simulink model "ES200A_CurrMeas"  (R2013b)
settings: Solver=FixedStepDiscrete  SolverMode=SingleTasking  StartTime=0.0  StopTime=1  FixedStep=0.000125  RelTol=1e-3
values from neighbouring files (symbols this model uses):
  ARCHGLBPRM_2PI_ULS_F32 = DataDict.Constant    [ES200A_CurrMeas_DataDict.m]
  CurrMeasEolGainMax = DataDict.Calibration    [ES200A_CurrMeas_DataDict.m]
  CurrMeasEolGainMin = DataDict.Calibration    [ES200A_CurrMeas_DataDict.m]
  CurrMeasEolGainNrOfSample = DataDict.Calibration    [ES200A_CurrMeas_DataDict.m]
  CurrMeasEolGainNumer = DataDict.Calibration    [ES200A_CurrMeas_DataDict.m]
  CurrMeasEolMaxMotVel = DataDict.Calibration    [ES200A_CurrMeas_DataDict.m]
  CurrMeasEolOffsHiBrdgVltgMin = DataDict.Calibration    [ES200A_CurrMeas_DataDict.m]
  CurrMeasEolOffsHiCmuOffs = DataDict.Calibration    [ES200A_CurrMeas_DataDict.m]
  CurrMeasEolOffsLoCmuOffs = DataDict.Calibration    [ES200A_CurrMeas_DataDict.m]
  CurrMeasEolOffsMax = DataDict.Calibration    [ES200A_CurrMeas_DataDict.m]
  CurrMeasEolOffsMin = DataDict.Calibration    [ES200A_CurrMeas_DataDict.m]
  CurrMeasEolOffsNrOfSample = DataDict.Calibration    [ES200A_CurrMeas_DataDict.m]
  CurrMeasEolTranCntrThd = DataDict.Calibration    [ES200A_CurrMeas_DataDict.m]
  CurrMeasMinRqrdPhaOnTi = DataDict.Calibration    [ES200A_CurrMeas_DataDict.m]
  CurrMeasMotAgCompuDly = DataDict.Calibration    [ES200A_CurrMeas_DataDict.m]
  CurrMeasMotCurrAdcVlyWrmIninMax = DataDict.Calibration    [ES200A_CurrMeas_DataDict.m]
  CurrMeasMotCurrAdcVlyWrmIninMin = DataDict.Calibration    [ES200A_CurrMeas_DataDict.m]
  CurrMeasNtc0x05DFailStep = DataDict.Calibration    [ES200A_CurrMeas_DataDict.m]
  CurrMeasNtc0x05DPassStep = DataDict.Calibration    [ES200A_CurrMeas_DataDict.m]
  CurrMeasNtc0x06DFailStep = DataDict.Calibration    [ES200A_CurrMeas_DataDict.m]
  CurrMeasNtc0x06DPassStep = DataDict.Calibration    [ES200A_CurrMeas_DataDict.m]
  DEGREES30_MOTRAD_F32 = DataDict.Constant    [ES200A_CurrMeas_DataDict.m]
  DIFOFFSRNGCHKMAX_VOLT_F32 = DataDict.Constant    [ES200A_CurrMeas_DataDict.m]
  ELECGLBPRM_IVTRCNT_CNT_U08 = DataDict.ConfigParam    [ES200A_CurrMeas_DataDict.m]
  ELECGLBPRM_STRTUPSTCURRMEASWRMININTESTSTRT_CNT_U08 = DataDict.Constant    [ES200A_CurrMeas_DataDict.m]
  FLTINJ_CURRMEAS_MOTCURRCORRDA = DataDict.Constant    [ES200A_CurrMeas_DataDict.m]
  FLTINJ_CURRMEAS_MOTCURRCORRDD = DataDict.Constant    [ES200A_CurrMeas_DataDict.m]
  FLTINJ_CURRMEAS_TESTOK = DataDict.Constant    [ES200A_CurrMeas_DataDict.m]
  MAXCURRCORRD_AMPR_F32 = DataDict.Constant    [ES200A_CurrMeas_DataDict.m]
  PhaABCMeasdOutOfRng = DataDict.NTC    [ES200A_CurrMeas_DataDict.m]
  PhaDEFMeasOutOfRng = DataDict.NTC    [ES200A_CurrMeas_DataDict.m]
  SysGlbPrmMotPoleCnt = DataDict.ImprtdCal    [ES200A_CurrMeas_DataDict.m]
libraries: simulink x10, FixdToFloat x1
(part 3 of 7)

== stateflow chart ES200A_CurrMeas/CurrMeas/CurrMeasPer1/Offset Calibration/Offset State Machine ==
  note: EolOffsSts
      |
      | 0 = Not Started
      | 1 = Started/In Process
      | 2 = Successful
      | 4  = Phase A, B, C EOL Calculated Gains are Out Of Range
      | 8  = Phase D, E, F EOL Calculated Gains are Out Of Range
      | 12 = Phase A, B, C, D, E, F EOL Calculated Gains are Out Of Range
      | 16  = VehSpd, VehSpdVld, condition not met
      | 32  = MotVelMrf condition not met
      | 64 = DiagcStsIvtr1Inactv and DiagcStsIvtr1Inactv both TRUE
  note: EolOffsOutOfRng = NTCNR_0X1EC
      | Parameters:
      |        Bit0Descr = 1 = 0000 0001 = Phase A, B, C EOL Calculated Offsets are Out Of Range
      |        Bit1Descr = 2 = 0000 0010 = Phase D, E, F EOL Calculated Offsets are Out Of Range
      |        Bit0Descr | Bit1Descr = 3 = 0000 0011 = Phase A, B, C, D, E, F EOL Calculated Offsets are Out Of Range
      |        Bit2Descr = 4 = 0000 0100 = VehSpd, VehSpdVld, condition not met
      |        Bit3Descr = 8 = 0000 1000 = MotVelMrf condition not met
      |        Bit3Descr = 16 = 0001 0000 = DiagcStsIvtr1Inactv and DiagcStsIvtr1Inactv both TRUE
  state MotCurrNtcSet = SetNtcSts(NTCNr,ParamBit,NTCSts,NTCDebStep) [function]
  note: EolOffsSts
      |
      | 0 = Not Started
      | 1 = Started/In Process
      | 2 = Successful
      | 4  = Phase A, B, C EOL Calculated Gains are Out Of Range
      | 8  = Phase D, E, F EOL Calculated Gains are Out Of Range
      | 12 = Phase A, B, C, D, E, F EOL Calculated Gains are Out Of Range
      | 16  = VehSpd, VehSpdVld, condition not met
      | 32  = MotVelMrf condition not met
      | 64 = DiagcStsIvtr1Inactv and DiagcStsIvtr1Inactv both TRUE
  note: EolOffsOutOfRng = NTCNR_0X1EC
      | Parameters:
      |        Bit0Descr = 1 = 0000 0001 = Phase A, B, C EOL Calculated Offsets are Out Of Range
      |        Bit1Descr = 2 = 0000 0010 = Phase D, E, F EOL Calculated Offsets are Out Of Range
      |
      |        Bit0Descr | Bit1Descr = 3 = 0000 0011 = Phase A, B, C, D, E, F EOL Calculated Offsets are Out Of Range
      |
      |        Bit2Descr = 4 = 0000 0100 = VehSpd, VehSpdVld, condition not met
      |        Bit3Descr = 8 = 0000 1000 = MotVelMrf condition not met
      |        Bit3Descr = 16 = 0001 0000 = DiagcStsIvtr1Inactv and DiagcStsIvtr1Inactv both TRUE
  state WrNvm [function]
  (default) -> (junction 307) : {EolOffsSts = EolOffsStsPrev;}
  (junction 307) -> (junction 233) [order 2] : {EolOffsSts = EolOffsStsPrev;}
  (junction 307) -> (junction 188) [order 1] : [EolOffsSts == 1]
  (junction 188) -> (junction 452) [order 1] : [(VehSpd <= ARCHGLBPRM_FLOATZEROTHD_ULS_F32 )...
      |  && (VehSpdVld == 1)]
  (junction 452) -> (junction 186) [order 1] : [(abs(MotVelMrf) <= CurrMeasEolMaxMotVel)]
  (junction 186) -> (junction 245) [order 2]
  (junction 245) -> (junction 263) [order 2]
  (junction 263) -> (junction 284) [order 2]
  (junction 284) -> (junction 294) [order 2]
  (junction 452) -> (junction 455) [order 2] : {CurrMeasMotCurrEolCalSt = MotCurrEolCalSt2.MCECS_CMDSAFEST;
      | MotCurrNtcSet = SetNtcSts(EolOffsOutOfRng, 8, 1, 0);
      | EolOffsSts = 32;}
  (junction 188) -> (junction 233) [order 2] : {CurrMeasMotCurrEolCalSt = MotCurrEolCalSt2.MCECS_CMDSAFEST;
      | MotCurrNtcSet = SetNtcSts(EolOffsOutOfRng, 4, 1, 0);
      | EolOffsSts = 16;}
  (junction 186) -> (junction 194) [order 1] : [(CurrMeasMotCurrEolCalStPrev == 0) || (CurrMeasMotCurrEolCalStPrev == 1)]
      | {CurrMeasMotCurrEolCalSt = MotCurrEolCalSt2.MCECS_OFFSCMDHI;}
  (junction 245) -> (junction 238) [order 1] : [CurrMeasMotCurrEolCalStPrev == MotCurrEolCalSt2.MCECS_OFFSCMDLO]
  (junction 263) -> (junction 256) [order 1] : [CurrMeasMotCurrEolCalStPrev == MotCurrEolCalSt2.MCECS_OFFSCMDZERO]
  (junction 284) -> (junction 395) [order 1] : [CurrMeasMotCurrEolCalStPrev == MotCurrEolCalSt2.MCECS_OFFSCMDEND && MotCurrEolOffsProcFlg != 1]
  (junction 294) -> (junction 295)
  (junction 395) -> (junction 414) [order 2] : {OffsRngChkABC = 1;}
  (junction 395) -> (junction 281) [order 1] : [DiagcStsIvtr1Inactv == 0]
  (junction 281) -> (junction 418) [order 2]
  (junction 418) -> (junction 434) : {OffsFltParam = 1;
      | OffsRngChkABC = 0;}
  (junction 281) -> (junction 414) [order 1] : [((MotCurrOffsHiAvrgA >= CurrMeasEolOffsMin) && (MotCurrOffsHiAvrgA <= CurrMeasEolOffsMax)) &&...
      | ((MotCurrOffsHiAvrgB >= CurrMeasEolOffsMin) && (MotCurrOffsHiAvrgB <= CurrMeasEolOffsMax)) &&...
      | ((MotCurrOffsHiAvrgC >= CurrMeasEolOffsMin) && (MotCurrOffsHiAvrgC <= CurrMeasEolOffsMax)) &&...
      | ((MotCurrOffsLoAvrgA >= CurrMeasEolOffsMin) && (MotCurrOffsLoAvrgA <= CurrMeasEolOffsMax)) &&...
      | ((MotCurrOffsLoAvrgB >= CurrMeasEolOffsMin) && (MotCurrOffsLoAvrgB <= CurrMeasEolOffsMax)) &&...
      | ((MotCurrOffsLoAvrgC >= CurrMeasEolOffsMin) && (MotCurrOffsLoAvrgC <= CurrMeasEolOffsMax))]
      |
      | {OffsRngChkABC = 1;}
  (junction 194) -> (junction 204) [order 2] : {CurrMeasEolTranCntr = CurrMeasEolTranCntrPrev + 1;}
  (junction 238) -> (junction 249) [order 2] : {CurrMeasEolTranCntr = CurrMeasEolTranCntrPrev + 1;}
  (junction 256) -> (junction 261) [order 2] : {CurrMeasEolTranCntr = CurrMeasEolTranCntrPrev + 1;}
  (junction 194) -> (junction 200) [order 1] : [CurrMeasEolTranCntr == CurrMeasEolTranCntrThd]
      |
      | {CurrMeasMotCurrSumA = CurrMeasMotCurrSumAPrev + MotCurrAdcVlyA;
      | CurrMeasMotCurrSumB = CurrMeasMotCurrSumBPrev + MotCurrAdcVlyB;
      | CurrMeasMotCurrSumC = CurrMeasMotCurrSumCPrev + MotCurrAdcVlyC;
      | CurrMeasMotCurrSumD = CurrMeasMotCurrSumDPrev + MotCurrAdcVlyD;
      | CurrMeasMotCurrSumE = CurrMeasMotCurrSumEPrev + MotCurrAdcVlyE;
      | CurrMeasMotCurrSumF = CurrMeasMotCurrSumFPrev + MotCurrAdcVlyF;
      | CurrMeasBrdgVltgSum = CurrMeasBrdgVltgSumPrev + BrdgVltg;
      |
      | CurrMeasEolAvrgCntr = CurrMeasEolAvrgCntrPrev + 1;}
  (junction 238) -> (junction 241) [order 1] : [CurrMeasEolTranCntr == CurrMeasEolTranCntrThd]
      |
      | {CurrMeasMotCurrSumA = CurrMeasMotCurrSumAPrev + MotCurrAdcVlyA;
      | CurrMeasMotCurrSumB = CurrMeasMotCurrSumBPrev + MotCurrAdcVlyB;
      | CurrMeasMotCurrSumC = CurrMeasMotCurrSumCPrev + MotCurrAdcVlyC;
      | CurrMeasMotCurrSumD = CurrMeasMotCurrSumDPrev + MotCurrAdcVlyD;
      | CurrMeasMotCurrSumE = CurrMeasMotCurrSumEPrev + MotCurrAdcVlyE;
      | CurrMeasMotCurrSumF = CurrMeasMotCurrSumFPrev + MotCurrAdcVlyF;
      |
      |
      | CurrMeasEolAvrgCntr = CurrMeasEolAvrgCntrPrev + 1;}
  (junction 256) -> (junction 254) [order 1] : [CurrMeasEolTranCntr == CurrMeasEolTranCntrThd]
      |
      | {CurrMeasMotCurrSumA = CurrMeasMotCurrSumAPrev + MotCurrAdcVlyA;
      | CurrMeasMotCurrSumB = CurrMeasMotCurrSumBPrev + MotCurrAdcVlyB;
      | CurrMeasMotCurrSumC = CurrMeasMotCurrSumCPrev + MotCurrAdcVlyC;
      | CurrMeasMotCurrSumD = CurrMeasMotCurrSumDPrev + MotCurrAdcVlyD;
      | CurrMeasMotCurrSumE = CurrMeasMotCurrSumEPrev + MotCurrAdcVlyE;
      | CurrMeasMotCurrSumF = CurrMeasMotCurrSumFPrev + MotCurrAdcVlyF;
      |
      |
      | CurrMeasEolAvrgCntr = CurrMeasEolAvrgCntrPrev + 1;}
  (junction 434) -> (junction 414)
  (junction 414) -> (junction 368)
  (junction 368) -> (junction 283) [order 2] : {OffsRngChkDEF = 1;}
  (junction 368) -> (junction 398) [order 1] : [DiagcStsIvtr2Inactv == 0 && ELECGLBPRM_IVTRCNT_CNT_U08 == 2]
  (junction 398) -> (junction 421) [order 2]
  (junction 421) -> (junction 436) : {OffsFltParam = OffsFltParam + 2
      | OffsRngChkDEF = 0;}
  (junction 398) -> (junction 283) [order 1] : [((MotCurrOffsHiAvrgD >= CurrMeasEolOffsMin) && (MotCurrOffsHiAvrgD <= CurrMeasEolOffsMax)) &&...
      | ((MotCurrOffsHiAvrgE >= CurrMeasEolOffsMin) && (MotCurrOffsHiAvrgE <= CurrMeasEolOffsMax)) &&...
      | ((MotCurrOffsHiAvrgF >= CurrMeasEolOffsMin) && (MotCurrOffsHiAvrgF <= CurrMeasEolOffsMax)) &&...
      | ((MotCurrOffsLoAvrgD >= CurrMeasEolOffsMin) && (MotCurrOffsLoAvrgD <= CurrMeasEolOffsMax)) &&...
      | ((MotCurrOffsLoAvrgE >= CurrMeasEolOffsMin) && (MotCurrOffsLoAvrgE <= CurrMeasEolOffsMax)) &&...
      | ((MotCurrOffsLoAvrgF >= CurrMeasEolOffsMin) && (MotCurrOffsLoAvrgF <= CurrMeasEolOffsMax))]
      |
      | {OffsRngChkDEF = 1;}
  (junction 436) -> (junction 283)
  (junction 283) -> (junction 439)
  (junction 200) -> (junction 204) [order 2]
  (junction 241) -> (junction 249) [order 2]
  (junction 254) -> (junction 261) [order 2]
  (junction 200) -> (junction 204) [order 1] : [CurrMeasEolAvrgCntr == CurrMeasEolOffsNrOfSample]
      |
      | {MotCurrOffsHiAvrgA = CurrMeasMotCurrSumA / CurrMeasEolOffsNrOfSample;
      | MotCurrOffsHiAvrgB = CurrMeasMotCurrSumB / CurrMeasEolOffsNrOfSample;
      | MotCurrOffsHiAvrgC = CurrMeasMotCurrSumC / CurrMeasEolOffsNrOfSample;
      | MotCurrOffsHiAvrgD = CurrMeasMotCurrSumD / CurrMeasEolOffsNrOfSample;
      | MotCurrOffsHiAvrgE = CurrMeasMotCurrSumE / CurrMeasEolOffsNrOfSample;
      | MotCurrOffsHiAvrgF = CurrMeasMotCurrSumF / CurrMeasEolOffsNrOfSample;
      | BrdgVltgAvrg  = CurrMeasBrdgVltgSum / CurrMeasEolOffsNrOfSample;
      | MotCurrEolOffsHiBrdgVltg = BrdgVltgAvrg * (CurrMeasEolOffsHiCmuOffs...
      |  - CurrMeasEolOffsLoCmuOffs);
      |
      | CurrMeasMotCurrEolCalSt = MotCurrEolCalSt2.MCECS_OFFSCMDLO;
      |
      | CurrMeasEolAvrgCntr = 0;
      | CurrMeasEolTranCntr = 0;
      |
      | CurrMeasMotCurrSumA = 0;
      | CurrMeasMotCurrSumB = 0;
      | CurrMeasMotCurrSumC = 0;
      | CurrMeasMotCurrSumD = 0;
      | CurrMeasMotCurrSumE = 0;
      | CurrMeasMotCurrSumF = 0;}
  (junction 241) -> (junction 249) [order 1] : [CurrMeasEolAvrgCntr == CurrMeasEolOffsNrOfSample]
      |
      | {MotCurrOffsLoAvrgA = CurrMeasMotCurrSumA / CurrMeasEolOffsNrOfSample;
      | MotCurrOffsLoAvrgB = CurrMeasMotCurrSumB / CurrMeasEolOffsNrOfSample;
      | MotCurrOffsLoAvrgC = CurrMeasMotCurrSumC / CurrMeasEolOffsNrOfSample;
      | MotCurrOffsLoAvrgD = CurrMeasMotCurrSumD / CurrMeasEolOffsNrOfSample;
      | MotCurrOffsLoAvrgE = CurrMeasMotCurrSumE / CurrMeasEolOffsNrOfSample;
      | MotCurrOffsLoAvrgF = CurrMeasMotCurrSumF / CurrMeasEolOffsNrOfSample;
      |
      |
      |
      |
      | CurrMeasMotCurrEolCalSt = MotCurrEolCalSt2.MCECS_OFFSCMDZERO;
      |
      | CurrMeasEolAvrgCntr = 0;
      | CurrMeasEolTranCntr = 0;
      |
      | CurrMeasMotCurrSumA = 0;
      | CurrMeasMotCurrSumB = 0;
      | CurrMeasMotCurrSumC = 0;
      | CurrMeasMotCurrSumD = 0;
      | CurrMeasMotCurrSumE = 0;
      | CurrMeasMotCurrSumF = 0;}
  (junction 254) -> (junction 261) [order 1] : [CurrMeasEolAvrgCntr == CurrMeasEolOffsNrOfSample]
      |
      | {MotCurrOffsZeroAvrgA = CurrMeasMotCurrSumA / CurrMeasEolOffsNrOfSample;
      | MotCurrOffsZeroAvrgB = CurrMeasMotCurrSumB / CurrMeasEolOffsNrOfSample;
      | MotCurrOffsZeroAvrgC = CurrMeasMotCurrSumC / CurrMeasEolOffsNrOfSample;
      | MotCurrOffsZeroAvrgD = CurrMeasMotCurrSumD / CurrMeasEolOffsNrOfSample;
      | MotCurrOffsZeroAvrgE = CurrMeasMotCurrSumE / CurrMeasEolOffsNrOfSample;
      | MotCurrOffsZeroAvrgF = CurrMeasMotCurrSumF / CurrMeasEolOffsNrOfSample;
      |
      |
      |
      |
      | CurrMeasMotCurrEolCalSt = MotCurrEolCalSt2.MCECS_OFFSCMDEND;
      |
      | CurrMeasEolAvrgCntr = 0;
      | CurrMeasEolTranCntr = 0;
      |
      | CurrMeasMotCurrSumA = 0;
      | CurrMeasMotCurrSumB = 0;
      | CurrMeasMotCurrSumC = 0;
      | CurrMeasMotCurrSumD = 0;
      | CurrMeasMotCurrSumE = 0;
      | CurrMeasMotCurrSumF = 0;}
  (junction 439) -> (junction 441) [order 2]
  (junction 441) -> (junction 417) : {
      | CurrMeasMotCurrEolCalSt = MotCurrEolCalSt2.MCECS_CMDSAFEST
      | MotCurrNtcSet = SetNtcSts(EolOffsOutOfRng, OffsFltParam, 1, 0);
      | EolOffsSts = OffsFltParam * 4;
      | CurrMeasEolAvrgCntr = 0;
      | CurrMeasEolTranCntr = 0;
      | }
  (junction 439) -> (junction 443) [order 1] : [OffsRngChkABC == 1 && OffsRngChkDEF == 1]
      | {
      | CurrMeasMotCurrEolCalSt = MotCurrEolCalSt2.MCECS_OFFSCMDEND;
      | CurrMeasEolAvrgCntr = 0;
      | CurrMeasEolTranCntr = 0;
      | }
  (junction 443) -> (junction 445) [order 2]
  (junction 445) -> (junction 422) : {
      | MotCurrNtcSet = SetNtcSts(EolOffsOutOfRng, 16, 1, 0);
      | EolOffsSts = 64;
      | CurrMeasMotCurrEolCalSt = MotCurrEolCalSt2.MCECS_CMDSAFEST;
      | }
  (junction 443) -> (junction 288) [order 1] : [(DiagcStsIvtr1Inactv == 0 || DiagcStsIvtr2Inactv == 0)]
      | {
      | MotCurrNtcSet = SetNtcSts(EolOffsOutOfRng, 0, 0, 0);
      | WrNvm();
      | MotCurrEolOffsProcFlg = 1;
      | EolOffsSts = 2;
      | }
  (junction 233) -> (junction 455)
  (junction 455) -> (junction 204)
  (junction 204) -> (junction 249)
  (junction 249) -> (junction 261)
  (junction 261) -> (junction 417)
  (junction 417) -> (junction 422)
  (junction 422) -> (junction 288)
  (junction 295) -> (junction 288)
  (junction 288) -> (junction 428)
  data: NTCNr function_input; ParamBit function_input; MotCurrNtcSet function_output; NTCSts function_input; NTCDebStep function_input; CurrMeasMotCurrEolCalSt output Enum: MotCurrEolCalSt2; EolOffsSts output uint8; MotCurrAdcVlyA input; MotCurrAdcVlyB input; MotCurrAdcVlyC input; MotCurrAdcVlyD input; MotCurrAdcVlyE input; MotCurrAdcVlyF input; BrdgVltg input; CurrMeasEolOffsNrOfSample input; CurrMeasEolOffsHiCmuOffs input; CurrMeasEolOffsLoCmuOffs input; CurrMeasEolOffsMax input; CurrMeasEolOffsMin input; BrdgVltgAvrg local double; BrdgVltgSum local double; MotCurrOffAvrgCntr local single; MotCurrSumHiA local single; MotCurrSumHiB local single; MotCurrSumHiC local single; MotCurrSumLoA local single; MotCurrSumLoB local single; MotCurrSumLoC local single; MotCurrSumZeroA local single; MotCurrSumZeroB local single; MotCurrSumZeroC local single; MotCurrOffsZeroAvrgA output single; MotCurrOffsZeroAvrgB output single; MotCurrOffsZeroAvrgC output single; MotCurrOffsZeroAvrgD output single; MotCurrOffsZeroAvrgE output single; MotCurrOffsZeroAvrgF output single; MotCurrEolOffsProcFlg output boolean; MotCurrEolOffsHiBrdgVltg output single; MotCurrOffsHiAvrgA output single; MotCurrOffsHiAvrgB output single; MotCurrOffsHiAvrgC output single; MotCurrOffsHiAvrgD output single; MotCurrOffsHiAvrgE output single; MotCurrOffsHiAvrgF output single; MotCurrSumHiD local single; MotCurrSumHiE local single; MotCurrSumHiF local single; MotCurrSumLoD local single; MotCurrSumLoE local single; MotCurrSumLoF local single; MotCurrSumZeroD local single; MotCurrSumZeroE local single; MotCurrSumZeroF local single; MotCurrOffsLoAvrgA output single; MotCurrNtcSet local single; NTC1EC constant single; CurrMeasEolMaxMotVel input; CurrMeasEolTranCntrThd input; MotVelMrf input; VehSpd input; VehSpdVld input; CurrMeasMotCurrEolCalStPrev input; EolOffsStsPrev input; ELECGLBPRM_IVTRCNT_CNT_U08 input; DiagcStsIvtr1Inactv input; DiagcStsIvtr2Inactv input; MotCurrOffsLoAvrgB output single; MotCurrOffsLoAvrgC output single; MotCurrOffsLoAvrgD output single; MotCurrOffsLoAvrgE output single; MotCurrOffsLoAvrgF output single; CurrMeasBrdgVltgSumPrev input; CurrMeasMotCurrSumAPrev input single; CurrMeasMotCurrSumBPrev input; CurrMeasMotCurrSumCPrev input; CurrMeasMotCurrSumDPrev input; CurrMeasMotCurrSumEPrev input; CurrMeasMotCurrSumFPrev input; CurrMeasBrdgVltgSum output single; CurrMeasMotCurrSumA output single; CurrMeasMotCurrSumB output single; CurrMeasMotCurrSumC output single; CurrMeasMotCurrSumD output single; CurrMeasMotCurrSumE output single; CurrMeasMotCurrSumF output single; CurrMeasEolTranCntrPrev input; CurrMeasEolAvrgCntrPrev input; CurrMeasEolTranCntr output uint8; CurrMeasEolAvrgCntr output uint16; EolOffsOutOfRng constant double; OffsRngChkABC local double; OffsRngChkDEF local double; OffsFltParam local double; ARCHGLBPRM_FLOATZEROTHD_ULS_F32 parameter

== system ES200A_CurrMeas/CurrMeas/CurrMeasEolOffsStsReq ==
  function : TriggerPort  TriggerType=function-call
  CopyRight2 : Subsystem  Description=|  mask(Copyright Information){none=on}
      | Copyright info block.                                               
      |                                                                     
      | Place copyright information at the top of every subsystem in design.
      mask prompts: none "No parameters"
      mask help: Place copyright information at the top of every subsystem in design.
      mask Display:
      | NxtrConf = 'Nexteer Confidential';
      | 
      | sys = bdroot; %handle for the current model ("system")
      | first = get_param(sys,'Created');
      | first = first(end-3:end);  %year is last four digits
      | 
      | last = get_param(sys,'LastModifiedDate');
      | if isempty(last)
      |     last = datestr(now,'yyyy');
      | else
      |     last = last(end-3:end);
      | end
      | 
      | if strcmp(first,last)
      |     fprintf('%s -- Copyright %s Nexteer',NxtrConf,first)
      | else
      |     fprintf('%s -- %s%s- %s Nexteer',NxtrConf,char(169),first,last)
      | end
  EolOffsSts : DataStoreRead  DataStoreName=EolOffsSts  DataStoreElements=EolOffsSts
  CurrMeasEolOffsSt : Outport
  wires:
  EolOffsSts/1 -> CurrMeasEolOffsSt/1

== system ES200A_CurrMeas/CurrMeas/CurrMeasGainReadReq ==
  function : TriggerPort
  CopyRight2 : Subsystem  Description=|  mask(Copyright Information){none=on}
      | Copyright info block.                                               
      |                                                                     
      | Place copyright information at the top of every subsystem in design.
      mask prompts: none "No parameters"
      mask help: Place copyright information at the top of every subsystem in design.
      mask Display:
      | NxtrConf = 'Nexteer Confidential';
      | 
      | sys = bdroot; %handle for the current model ("system")
      | first = get_param(sys,'Created');
      | first = first(end-3:end);  %year is last four digits
      | 
      | last = get_param(sys,'LastModifiedDate');
      | if isempty(last)
      |     last = datestr(now,'yyyy');
      | else
      |     last = last(end-3:end);
      | end
      | 
      | if strcmp(first,last)
      |     fprintf('%s -- Copyright %s Nexteer',NxtrConf,first)
      | else
      |     fprintf('%s -- %s%s- %s Nexteer',NxtrConf,char(169),first,last)
      | end
  CurrMeasEolGainCalSet : DataStoreRead  DataStoreName=CurrMeasEolGainCalSet  DataStoreElements=CurrMeasEolGainCalSet.CurrMeasMotCurrEolGainA#CurrMeasEolGainCalSet.CurrMeasMotCurrEolGainB#CurrMeasEolGainCalSet.CurrMeasMotCurrEolGainC#CurrMeasEolGainCalSet.CurrMeasMotCurrEolGainD#CurrMeasEolGainCalSet.CurrMeasMotCurrEolGainE#CurrMeasEolGainCalSet.CurrMeasMotCurrEolGainF
  CurrMeasMotCurrGainA_ArgOut : Outport  RequirementInfo={} %GIDa_c0bd7469_2a75_4ce8_87e1_f0e93a31fe96
  CurrMeasMotCurrGainB_ArgOut : Outport  RequirementInfo={} %GIDa_1bb15bff_a71c_44aa_82e2_2ad06761edd2  Port=2
  CurrMeasMotCurrGainC_ArgOut : Outport  RequirementInfo={} %GIDa_44ce3810_b044_40e2_a3c4_2ff9160dcac8  Port=3
  CurrMeasMotCurrGainD_ArgOut : Outport  RequirementInfo={} %GIDa_a35aebc1_14fb_4199_815e_57d26626d03d  Port=4
  CurrMeasMotCurrGainE_ArgOut : Outport  RequirementInfo={} %GIDa_c5746494_b09e_49e9_84e1_76a43de95384  Port=5
  CurrMeasMotCurrGainF_ArgOut : Outport  RequirementInfo={} %GIDa_d57b5961_0392_456f_a038_0afe8120a51f  Port=6
  wires:
  CurrMeasEolGainCalSet/1 -> CurrMeasMotCurrGainA_ArgOut/1
  CurrMeasEolGainCalSet/2 -> CurrMeasMotCurrGainB_ArgOut/1
  CurrMeasEolGainCalSet/3 -> CurrMeasMotCurrGainC_ArgOut/1
  CurrMeasEolGainCalSet/4 -> CurrMeasMotCurrGainD_ArgOut/1
  CurrMeasEolGainCalSet/5 -> CurrMeasMotCurrGainE_ArgOut/1
  CurrMeasEolGainCalSet/6 -> CurrMeasMotCurrGainF_ArgOut/1

== system ES200A_CurrMeas/CurrMeas/CurrMeasGainWrReq ==
  CurrMeasMotCurrGainA_ArgIn : Inport  RequirementInfo={} %GIDa_c425d1ca_be7a_40e5_bba5_162e843ab10f  OutDataTypeStr=single
  CurrMeasMotCurrGainB_ArgIn : Inport  RequirementInfo={} %GIDa_bd7d1dd6_00d8_4c0e_b958_cd79b1c62016  Port=2  OutDataTypeStr=single
  CurrMeasMotCurrGainC_ArgIn : Inport  RequirementInfo={} %GIDa_442e802f_e2c7_406d_b1fc_b8f70d0353c6  Port=3  OutDataTypeStr=single
  CurrMeasMotCurrGainD_ArgIn : Inport  RequirementInfo={} %GIDa_a6de7fab_9a7f_4a18_932a_688a0ad19497  Port=4  OutDataTypeStr=single
  CurrMeasMotCurrGainE_ArgIn : Inport  RequirementInfo={} %GIDa_58241980_a2a0_46cb_8faf_4af881b5bc84  Port=5  OutDataTypeStr=single
  CurrMeasMotCurrGainF_ArgIn : Inport  RequirementInfo={} %GIDa_7c5d0880_7e38_46fb_95a6_ac4fe6cd7a27  Port=6  OutDataTypeStr=single
  function : TriggerPort
  Constant1 : Constant  Value=CurrMeasEolGainMax  OutDataTypeStr=single
  Constant3 : Constant  Value=CurrMeasEolGainMin  OutDataTypeStr=single
  CopyRight2 : Subsystem  Description=|  mask(Copyright Information){none=on}
      | Copyright info block.                                               
      |                                                                     
      | Place copyright information at the top of every subsystem in design.
      mask prompts: none "No parameters"
      mask help: Place copyright information at the top of every subsystem in design.
      mask Display:
      | NxtrConf = 'Nexteer Confidential';
      | 
      | sys = bdroot; %handle for the current model ("system")
      | first = get_param(sys,'Created');
      | first = first(end-3:end);  %year is last four digits
      | 
      | last = get_param(sys,'LastModifiedDate');
      | if isempty(last)
      |     last = datestr(now,'yyyy');
      | else
      |     last = last(end-3:end);
      | end
      | 
      | if strcmp(first,last)
      |     fprintf('%s -- Copyright %s Nexteer',NxtrConf,first)
      | else
      |     fprintf('%s -- %s%s- %s Nexteer',NxtrConf,char(169),first,last)
      | end
  IF : Subsystem  RequirementInfo={'linktype_rmi_doors' '000089bc (/ESG Group/FDD Module Requirements/EA4 Specific/ES200A_CurrMeas)' '#ES200A_291' 'true' 'REQ: ES200A_291' '' } %GIDa_4876ff6b_f5fc_4b95_bbc0_660fa9cc47c9  TreatAsAtomicUnit=on
  If1 : If  RequirementInfo={'linktype_rmi_doors' '000089bc (/ESG Group/FDD Module Requirements/EA4 Specific/ES200A_CurrMeas)' '#ES200A_291' 'true' 'REQ: ES200A_291' '' } %GIDa_99201fd8_db84_4d56_a868_77c34be46a9e  NumInputs=8  IfExpression=(u1 <= u3 & u3 <= u2) & (u1 <= u4 & u4 <= u2) & (u1 <= u5 & u5 <= u2) & (u1 <= u6 & u6 <= u2) & (u1 <= u7 & u7 <= u2) & (u1 <= u8 & u8 <= u2)
  Merge : Merge
  "else " : Subsystem  TreatAsAtomicUnit=on
  CurrMeasGainWrReqSts : Outport  RequirementInfo={} %GIDa_00298d30_c602_4e54_ac9c_fe9e46cb7e08
  wires:
  If1/1 -> IF/Action
  Constant3/1 -> If1/1
  Constant1/1 -> If1/2
  CurrMeasMotCurrGainC_ArgIn/1 -> IF/3(CurrMeasMotCurrGainC_ArgIn), If1/5  "CurrMeasMotCurrGainC_ArgIn"
  CurrMeasMotCurrGainD_ArgIn/1 -> IF/4(CurrMeasMotCurrGainD_ArgIn), If1/6  "CurrMeasMotCurrGainD_ArgIn"
  CurrMeasMotCurrGainB_ArgIn/1 -> IF/2(CurrMeasMotCurrGainB_ArgIn), If1/4  "CurrMeasMotCurrGainB_ArgIn"
  CurrMeasMotCurrGainE_ArgIn/1 -> IF/5(CurrMeasMotCurrGainE_ArgIn), If1/7  "CurrMeasMotCurrGainE_ArgIn"
  CurrMeasMotCurrGainA_ArgIn/1 -> IF/1(CurrMeasMotCurrGainA_ArgIn), If1/3  "CurrMeasMotCurrGainA_ArgIn"
  CurrMeasMotCurrGainF_ArgIn/1 -> IF/6(CurrMeasMotCurrGainF_ArgIn), If1/8  "CurrMeasMotCurrGainF_ArgIn"
  If1/2 -> "else "/Action
  Merge/1 -> CurrMeasGainWrReqSts/1
  "else "/1(CurrMeasGainWrReqSts) -> Merge/1
  IF/1(CurrMeasGainWrReqSts) -> Merge/2

== system ES200A_CurrMeas/CurrMeas/CurrMeasInit1 ==
  CurrMeasEolOffsHiBrdgVltgMin : Inport
  Trigger : TriggerPort  TriggerType=function-call  PortDimensions=1
  CopyRight2 : Subsystem  Description=|  mask(Copyright Information){none=on}
      | Copyright info block.                                               
      |                                                                     
      | Place copyright information at the top of every subsystem in design.
      mask prompts: none "No parameters"
      mask help: Place copyright information at the top of every subsystem in design.
      mask Display:
      | NxtrConf = 'Nexteer Confidential';
      | 
      | sys = bdroot; %handle for the current model ("system")
      | first = get_param(sys,'Created');
      | first = first(end-3:end);  %year is last four digits
      | 
      | last = get_param(sys,'LastModifiedDate');
      | if isempty(last)
      |     last = datestr(now,'yyyy');
      | else
      |     last = last(end-3:end);
      | end
      | 
      | if strcmp(first,last)
      |     fprintf('%s -- Copyright %s Nexteer',NxtrConf,first)
      | else
      |     fprintf('%s -- %s%s- %s Nexteer',NxtrConf,char(169),first,last)
      | end
  CurrMeasEolOffsCalSet : DataStoreRead  RequirementInfo={'linktype_rmi_doors' '000089bc (/ESG Group/FDD Module Requirements/EA4 Specific/ES200A_CurrMeas)' '#ES200A_280' 'true' 'REQ: ES200A_280' '' } %GIDa_5b13b3a8_fa13_45cc_ae87_baf34a1014a6  DataStoreName=CurrMeasEolOffsCalSet  DataStoreElements=CurrMeasEolOffsCalSet.CurrMeasMotCurrEolOffsDifA#CurrMeasEolOffsCalSet.CurrMeasMotCurrEolOffsDifB#CurrMeasEolOffsCalSet.CurrMeasMotCurrEolOffsDifC#CurrMeasEolOffsCalSet.CurrMeasEolOffsHiBrdgVltg#CurrMeasEolOffsCalSet.CurrMeasMotCurrEolOffsDifD#CurrMeasEolOffsCalSet.CurrMeasMotCurrEolOffsDifE#CurrMeasEolOffsCalSet.CurrMeasMotCurrEolOffsDifF
  If : If  NumInputs=2  IfExpression=u1>u2
  If Action Subsystem : Subsystem  TreatAsAtomicUnit=on
  If Action Subsystem1 : Subsystem  TreatAsAtomicUnit=on
  Merge{1..6} (6 alike) : Merge
  MotCurrOffsDeltaA : Outport
  MotCurrOffsDeltaB : Outport  Port=2
  MotCurrOffsDeltaC : Outport  Port=3
  MotCurrOffsDeltaD : Outport  Port=4
  MotCurrOffsDeltaE : Outport  Port=5
  MotCurrOffsDeltaF : Outport  Port=6
  wires:
  CurrMeasEolOffsHiBrdgVltgMin/1 -> If/2
  If/1 -> If Action Subsystem/Action
  If/2 -> If Action Subsystem1/Action
  If Action Subsystem/1(MotCurrOffsDeltaA) -> Merge1/1
  If Action Subsystem/2(MotCurrOffsDeltaB) -> Merge2/1
  If Action Subsystem/3(MotCurrOffsDeltaC) -> Merge3/1
  If Action Subsystem/4(MotCurrOffsDeltaD) -> Merge4/1
  If Action Subsystem/5(MotCurrOffsDeltaE) -> Merge5/1
  If Action Subsystem/6(MotCurrOffsDeltaF) -> Merge6/1
  If Action Subsystem1/1(MotCurrOffsDeltaA) -> Merge1/2
  If Action Subsystem1/2(MotCurrOffsDeltaB) -> Merge2/2
  If Action Subsystem1/3(MotCurrOffsDeltaC) -> Merge3/2
  If Action Subsystem1/4(MotCurrOffsDeltaD) -> Merge4/2
  If Action Subsystem1/5(MotCurrOffsDeltaE) -> Merge5/2
  If Action Subsystem1/6(MotCurrOffsDeltaF) -> Merge6/2
  Merge1/1 -> MotCurrOffsDeltaA/1
  Merge2/1 -> MotCurrOffsDeltaB/1
  Merge3/1 -> MotCurrOffsDeltaC/1
  Merge4/1 -> MotCurrOffsDeltaD/1
  Merge5/1 -> MotCurrOffsDeltaE/1
  Merge6/1 -> MotCurrOffsDeltaF/1
  CurrMeasEolOffsCalSet/5 -> If Action Subsystem/5(MotCurrEolOffsDifD)
  CurrMeasEolOffsCalSet/3 -> If Action Subsystem/3(MotCurrEolOffsDifC)
  CurrMeasEolOffsCalSet/6 -> If Action Subsystem/6(MotCurrEolOffsDifE)
  CurrMeasEolOffsCalSet/1 -> If Action Subsystem/1(MotCurrEolOffsDifA)
  CurrMeasEolOffsCalSet/2 -> If Action Subsystem/2(MotCurrEolOffsDifB)
  CurrMeasEolOffsCalSet/7 -> If Action Subsystem/7(MotCurrEolOffsDifF)
  CurrMeasEolOffsCalSet/4 -> If/1, If Action Subsystem/4(CurrMeasEolOffsHiBrdgVltg)

== system ES200A_CurrMeas/CurrMeas/CurrMeasOffsReadReq ==
  function : TriggerPort
  CopyRight2 : Subsystem  Description=|  mask(Copyright Information){none=on}
      | Copyright info block.                                               
      |                                                                     
      | Place copyright information at the top of every subsystem in design.
      mask prompts: none "No parameters"
      mask help: Place copyright information at the top of every subsystem in design.
      mask Display:
      | NxtrConf = 'Nexteer Confidential';
      | 
      | sys = bdroot; %handle for the current model ("system")
      | first = get_param(sys,'Created');
      | first = first(end-3:end);  %year is last four digits
      | 
      | last = get_param(sys,'LastModifiedDate');
      | if isempty(last)
      |     last = datestr(now,'yyyy');
      | else
      |     last = last(end-3:end);
      | end
      | 
      | if strcmp(first,last)
      |     fprintf('%s -- Copyright %s Nexteer',NxtrConf,first)
      | else
      |     fprintf('%s -- %s%s- %s Nexteer',NxtrConf,char(169),first,last)
      | end
  CurrMeasEolOffsCalSet : DataStoreRead  RequirementInfo={'linktype_rmi_doors' '000089bc (/ESG Group/FDD Module Requirements/EA4 Specific/ES200A_CurrMeas)' '#ES200A_280' 'true' 'REQ: ES200A_280' '' } %GIDa_8cba0bc8_e323_4e1f_8e86_73dafe0bba1d  DataStoreName=CurrMeasEolOffsCalSet  DataStoreElements=CurrMeasEolOffsCalSet.CurrMeasEolOffsHiBrdgVltg#CurrMeasEolOffsCalSet.CurrMeasMotCurrEolOffsDifA#CurrMeasEolOffsCalSet.CurrMeasMotCurrEolOffsDifB#CurrMeasEolOffsCalSet.CurrMeasMotCurrEolOffsDifC#CurrMeasEolOffsCalSet.CurrMeasMotCurrEolOffsDifD#CurrMeasEolOffsCalSet.CurrMeasMotCurrEolOffsDifE#CurrMeasEolOffsCalSet.CurrMeasMotCurrEolOffsDifF#CurrMeasEolOffsCalSet.CurrMeasMotCurrOffsLoAvrgA#CurrMeasEolOffsCalSet.CurrMeasMotCurrOffsLoAvrgB#CurrMeasEolOffsCalSet.CurrMeasMotCurrOffsLoAvrgC#CurrMeasEolOffsCalSet.CurrMeasMotCurrOffsLoAvrgD#CurrMeasEolOffsCalSet.CurrMeasMotCurrOffsLoAvrgE#CurrMeasEolOffsCalSet.CurrMeasMotCurrOffsLoAvrgF
  CurrMeasEolOffsHiBrdgVltg_ArgOut : Outport  RequirementInfo={} %GIDa_c2b0fe9d_3793_43b9_8623_9e15e29718c9
  CurrMeasMotCurrOffsDifA_ArgOut : Outport  RequirementInfo={} %GIDa_06880cd0_b3c9_4dac_a20b_1d769ce6ab3e  Port=2
  CurrMeasMotCurrOffsDifB_ArgOut : Outport  RequirementInfo={} %GIDa_89879a61_0bc4_4d01_9a03_1b0943ab4d4d  Port=3
  CurrMeasMotCurrOffsDifC_ArgOut : Outport  RequirementInfo={} %GIDa_a1432bf3_c07e_4e99_b270_4232122d4772  Port=4
  CurrMeasMotCurrOffsDifD_ArgOut : Outport  RequirementInfo={} %GIDa_3df17fd6_11a6_4a3b_a21f_0f2b4386103a  Port=5
  CurrMeasMotCurrOffsDifE_ArgOut : Outport  RequirementInfo={} %GIDa_8531bc1c_851e_4a5c_bd1a_ff758ac49903  Port=6
  CurrMeasMotCurrOffsDifF_ArgOut : Outport  RequirementInfo={} %GIDa_d9d2e87e_a616_4443_9719_46d0ee8ea0d2  Port=7
  CurrMeasMotCurrOffsLoAvrgA_ArgOut : Outport  RequirementInfo={} %GIDa_c5194a62_6435_4295_b125_fb72e5f95c25  Port=8
  CurrMeasMotCurrOffsLoAvrgB_ArgOut : Outport  RequirementInfo={} %GIDa_76f08b3f_5cc7_46f2_a183_091f4f2205e6  Port=9
  CurrMeasMotCurrOffsLoAvrgC_ArgOut : Outport  RequirementInfo={} %GIDa_b1bbc18a_9d6a_4672_bdc3_0bccd18a5fef  Port=10
  CurrMeasMotCurrOffsLoAvrgD_ArgOut : Outport  RequirementInfo={} %GIDa_3f8d0b0a_e576_41bf_81a1_80b77bc69872  Port=11
  CurrMeasMotCurrOffsLoAvrgE_ArgOut : Outport  RequirementInfo={} %GIDa_06d47c59_3406_4ddb_96f7_958a6ee8ee04  Port=12
  CurrMeasMotCurrOffsLoAvrgF_ArgOut : Outport  RequirementInfo={} %GIDa_8b869263_e1b4_42a0_8921_d65f6bf7b80b  Port=13
  wires:
  CurrMeasEolOffsCalSet/1 -> CurrMeasEolOffsHiBrdgVltg_ArgOut/1
  CurrMeasEolOffsCalSet/2 -> CurrMeasMotCurrOffsDifA_ArgOut/1
  CurrMeasEolOffsCalSet/3 -> CurrMeasMotCurrOffsDifB_ArgOut/1
  CurrMeasEolOffsCalSet/4 -> CurrMeasMotCurrOffsDifC_ArgOut/1
  CurrMeasEolOffsCalSet/5 -> CurrMeasMotCurrOffsDifD_ArgOut/1
  CurrMeasEolOffsCalSet/6 -> CurrMeasMotCurrOffsDifE_ArgOut/1
  CurrMeasEolOffsCalSet/7 -> CurrMeasMotCurrOffsDifF_ArgOut/1
  CurrMeasEolOffsCalSet/8 -> CurrMeasMotCurrOffsLoAvrgA_ArgOut/1
  CurrMeasEolOffsCalSet/9 -> CurrMeasMotCurrOffsLoAvrgB_ArgOut/1
  CurrMeasEolOffsCalSet/10 -> CurrMeasMotCurrOffsLoAvrgC_ArgOut/1
  CurrMeasEolOffsCalSet/11 -> CurrMeasMotCurrOffsLoAvrgD_ArgOut/1
  CurrMeasEolOffsCalSet/12 -> CurrMeasMotCurrOffsLoAvrgE_ArgOut/1
  CurrMeasEolOffsCalSet/13 -> CurrMeasMotCurrOffsLoAvrgF_ArgOut/1

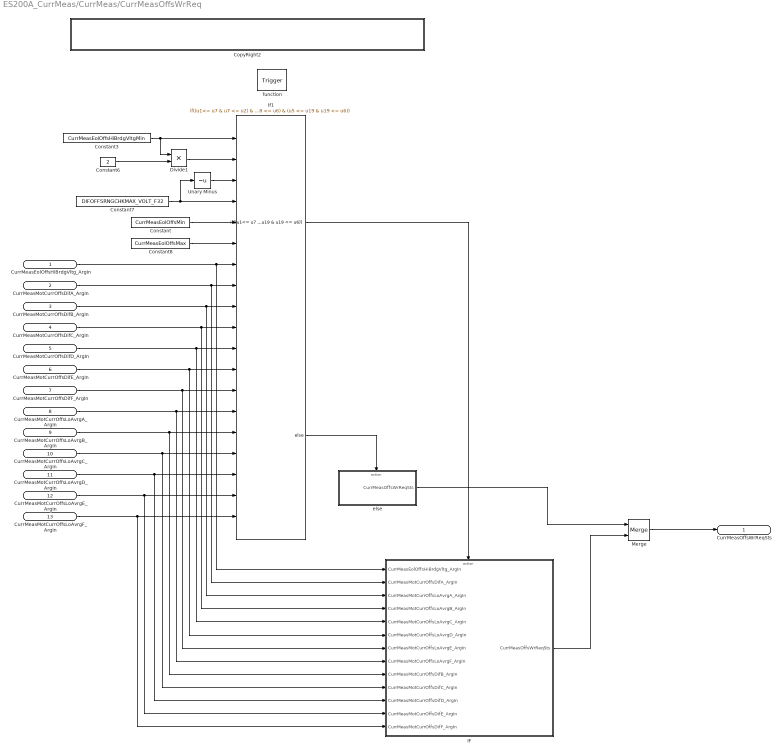
== system ES200A_CurrMeas/CurrMeas/CurrMeasOffsWrReq ==
  CurrMeasEolOffsHiBrdgVltg_ArgIn : Inport  RequirementInfo={} %GIDa_20319714_70ba_40b8_83d5_5be49dcbe6c0  OutDataTypeStr=single
  CurrMeasMotCurrOffsDifA_ArgIn : Inport  RequirementInfo={} %GIDa_567da3a1_0d48_4934_8feb_e936b086fb7e  Port=2  OutDataTypeStr=single
  CurrMeasMotCurrOffsDifB_ArgIn : Inport  RequirementInfo={} %GIDa_d0ed0aa3_f35f_4142_b108_d1399608bd37  Port=3  OutDataTypeStr=single
  CurrMeasMotCurrOffsDifC_ArgIn : Inport  RequirementInfo={} %GIDa_333f9d57_9630_4d9a_bf0a_758004fd24d5  Port=4  OutDataTypeStr=single
  CurrMeasMotCurrOffsDifD_ArgIn : Inport  RequirementInfo={} %GIDa_75702a95_bde2_4d36_99b5_54163b4c7153  Port=5  OutDataTypeStr=single
  CurrMeasMotCurrOffsDifE_ArgIn : Inport  RequirementInfo={} %GIDa_d5c11ab6_7fa1_4a01_9aa2_8e70eb92dca0  Port=6  OutDataTypeStr=single
  CurrMeasMotCurrOffsDifF_ArgIn : Inport  RequirementInfo={} %GIDa_93b2894a_d1d3_46df_b4ef_6d97a088df41  Port=7  OutDataTypeStr=single
  CurrMeasMotCurrOffsLoAvrgA_ArgIn : Inport  RequirementInfo={} %GIDa_d3fc1696_9b01_4bfe_ae5b_43ed0baf9797  Port=8  OutDataTypeStr=single
  CurrMeasMotCurrOffsLoAvrgB_ArgIn : Inport  RequirementInfo={} %GIDa_e3286a61_69ab_4ddc_b4c3_7297f20485dd  Port=9  OutDataTypeStr=single
  CurrMeasMotCurrOffsLoAvrgC_ArgIn : Inport  RequirementInfo={} %GIDa_d0fb0236_0795_4629_a145_caa3ab5bd346  Port=10  OutDataTypeStr=single
  CurrMeasMotCurrOffsLoAvrgD_ArgIn : Inport  RequirementInfo={} %GIDa_8377999d_f727_4278_a09a_19b59b7325e4  Port=11  OutDataTypeStr=single
  CurrMeasMotCurrOffsLoAvrgE_ArgIn : Inport  RequirementInfo={} %GIDa_308508b2_c858_4477_ae29_a4055a9a0165  Port=12  OutDataTypeStr=single
  CurrMeasMotCurrOffsLoAvrgF_ArgIn : Inport  RequirementInfo={} %GIDa_00179445_133e_4a7c_829d_b4552183115d  Port=13  OutDataTypeStr=single
  function : TriggerPort
  Constant : Constant  Value=CurrMeasEolOffsMin
  Constant3 : Constant  Value=CurrMeasEolOffsHiBrdgVltgMin  OutDataTypeStr=single
  Constant6 : Constant  Value=2  OutDataTypeStr=single
  Constant7 : Constant  Value=DIFOFFSRNGCHKMAX_VOLT_F32  OutDataTypeStr=single
  Constant8 : Constant  Value=CurrMeasEolOffsMax
  CopyRight2 : Subsystem  Description=|  mask(Copyright Information){none=on}
      | Copyright info block.                                               
      |                                                                     
      | Place copyright information at the top of every subsystem in design.
      mask prompts: none "No parameters"
      mask help: Place copyright information at the top of every subsystem in design.
      mask Display:
      | NxtrConf = 'Nexteer Confidential';
      | 
      | sys = bdroot; %handle for the current model ("system")
      | first = get_param(sys,'Created');
      | first = first(end-3:end);  %year is last four digits
      | 
      | last = get_param(sys,'LastModifiedDate');
      | if isempty(last)
      |     last = datestr(now,'yyyy');
      | else
      |     last = last(end-3:end);
      | end
      | 
      | if strcmp(first,last)
      |     fprintf('%s -- Copyright %s Nexteer',NxtrConf,first)
      | else
      |     fprintf('%s -- %s%s- %s Nexteer',NxtrConf,char(169),first,last)
      | end
  Divide1 : Product  Inputs=**  OutDataTypeStr=single
  IF : Subsystem  RequirementInfo={'linktype_rmi_doors' '000089bc (/ESG Group/FDD Module Requirements/EA4 Specific/ES200A_CurrMeas)' '#ES200A_280' 'true' 'REQ: ES200A_280' '' } %GIDa_94ca970e_96f2_476d_8160_5cb99576e311  TreatAsAtomicUnit=on
  If1 : If  RequirementInfo={'linktype_rmi_doors' '000089bc (/ESG Group/FDD Module Requirements/EA4 Specific/ES200A_CurrMeas)' '#ES200A_280' 'true' 'REQ: ES200A_280' '' } %GIDa_9a24cfae_c3f3_4b93_a488_aa733d7ab090  NumInputs=19  IfExpression=(u1<= u7 & u7 <= u2) & (u3 <= u8 & u8 <= u4) & (u3 <= u9 & u9 <= u4) & (u3 <= u10 & u10 < u4) & (u3 <= u11 & u11 <= u4) & (u3 <= u12 & u12 <= u4) & (u3 <= u13 & u13 <= u4) & (u5 <= u14 & u14 <= u6) & (u5 <= u15 & u15 <= u6) & (u5 <= u16 & u16 <= u6) & (u5 <= u17 & u17 <= u6) & (u5 <= u18 & u18 <= u6) & (u5 <= u19 & u19 <= u6)
  Merge : Merge
  Unary Minus : UnaryMinus
  "else " : Subsystem  TreatAsAtomicUnit=on
  CurrMeasOffsWrReqSts : Outport  RequirementInfo={} %GIDa_e38a5dae_03c2_4788_8854_754d30bf24dd
  wires:
  Constant3/1 -> If1/1, Divide1/1
  Constant6/1 -> Divide1/2
  Unary Minus/1 -> If1/3
  Constant7/1 -> Unary Minus/1, If1/4
  Constant8/1 -> If1/6
  Constant/1 -> If1/5
  CurrMeasEolOffsHiBrdgVltg_ArgIn/1 -> IF/1(CurrMeasEolOffsHiBrdgVltg_ArgIn), If1/7
  CurrMeasMotCurrOffsDifA_ArgIn/1 -> IF/2(CurrMeasMotCurrOffsDifA_ArgIn), If1/8
  CurrMeasMotCurrOffsDifB_ArgIn/1 -> IF/3(CurrMeasMotCurrOffsLoAvrgA_ArgIn), If1/9
  CurrMeasMotCurrOffsDifC_ArgIn/1 -> IF/4(CurrMeasMotCurrOffsLoAvrgB_ArgIn), If1/10
  CurrMeasMotCurrOffsDifD_ArgIn/1 -> IF/5(CurrMeasMotCurrOffsLoAvrgC_ArgIn), If1/11
  CurrMeasMotCurrOffsDifE_ArgIn/1 -> IF/6(CurrMeasMotCurrOffsLoAvrgD_ArgIn), If1/12
  CurrMeasMotCurrOffsLoAvrgA_ArgIn/1 -> IF/8(CurrMeasMotCurrOffsLoAvrgF_ArgIn), If1/14
  CurrMeasMotCurrOffsLoAvrgB_ArgIn/1 -> IF/9(CurrMeasMotCurrOffsDifB_ArgIn), If1/15
  CurrMeasMotCurrOffsLoAvrgE_ArgIn/1 -> IF/12(CurrMeasMotCurrOffsDifE_ArgIn), If1/18
  CurrMeasMotCurrOffsLoAvrgF_ArgIn/1 -> IF/13(CurrMeasMotCurrOffsDifF_ArgIn), If1/19
  CurrMeasMotCurrOffsLoAvrgC_ArgIn/1 -> IF/10(CurrMeasMotCurrOffsDifC_ArgIn), If1/16
  If1/1 -> IF/Action
  CurrMeasMotCurrOffsDifF_ArgIn/1 -> IF/7(CurrMeasMotCurrOffsLoAvrgE_ArgIn), If1/13
  CurrMeasMotCurrOffsLoAvrgD_ArgIn/1 -> IF/11(CurrMeasMotCurrOffsDifD_ArgIn), If1/17
  If1/2 -> "else "/Action
  Divide1/1 -> If1/2
  Merge/1 -> CurrMeasOffsWrReqSts/1
  "else "/1(CurrMeasOffsWrReqSts) -> Merge/1
  IF/1(CurrMeasOffsWrReqSts) -> Merge/2

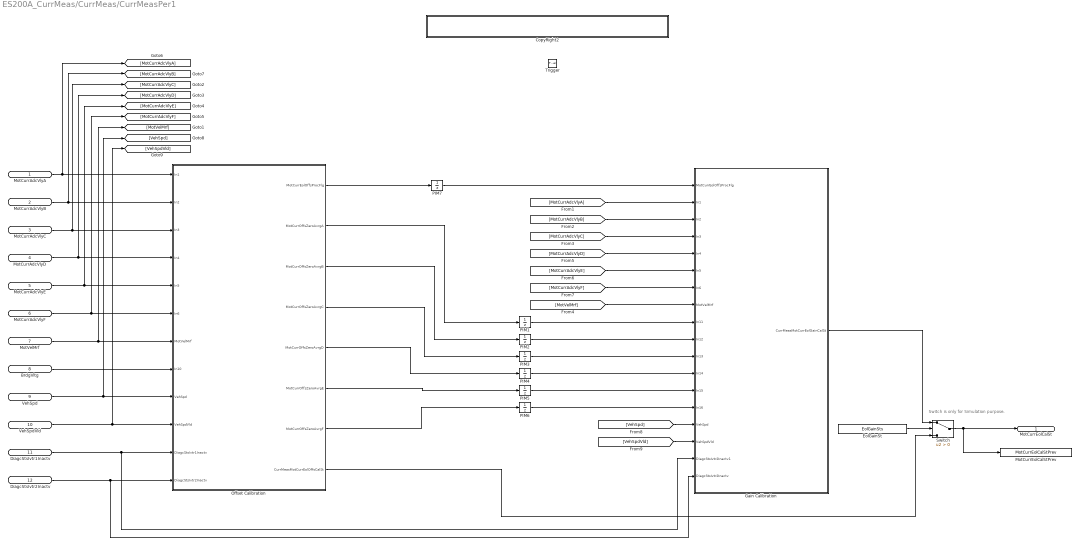
== system ES200A_CurrMeas/CurrMeas/CurrMeasPer1 ==
  note: Switch is only for Simulation purpose.
  MotCurrAdcVlyA : Inport  RequirementInfo={} %GIDa_d6fdc2a5_c36f_4862_a3e7_4b336023a3c4  OutDataTypeStr=single
  MotCurrAdcVlyB : Inport  RequirementInfo={} %GIDa_329e32be_6008_45fd_bd72_340d7ae8c1b5  Port=2  OutDataTypeStr=single
  MotCurrAdcVlyC : Inport  RequirementInfo={} %GIDa_746c9616_e976_40d7_b54a_823dc364fe71  Port=3  OutDataTypeStr=single
  MotCurrAdcVlyD : Inport  RequirementInfo={} %GIDa_4b06763f_6209_4b7f_9565_5c5d2daca03a  Port=4  OutDataTypeStr=single
  MotCurrAdcVlyE : Inport  RequirementInfo={} %GIDa_3a5b9e65_aa66_45a4_8818_13580434b978  Port=5  OutDataTypeStr=single
  MotCurrAdcVlyF : Inport  RequirementInfo={} %GIDa_3a4efe1c_5ef6_4746_95ad_6493d8eca6d1  Port=6  OutDataTypeStr=single
  MotVelMrf : Inport  RequirementInfo={} %GIDa_3549e207_a5ba_4370_a041_76429f88a9dd  Port=7  OutDataTypeStr=single
  BrdgVltg : Inport  RequirementInfo={} %GIDa_3ee59834_071a_42af_a764_5aee71a021cf  Port=8  OutDataTypeStr=single
  VehSpd : Inport  RequirementInfo={} %GIDa_3dad792b_6867_498d_8cf5_08b87633e71b  Port=9
  VehSpdVld : Inport  RequirementInfo={} %GIDa_79ad4a0e_1634_487e_a0d4_030cd7a6c3f9  Port=10
  DiagcStsIvtr1Inactv : Inport  RequirementInfo={} %GIDa_c8c114ff_24fe_44c5_88f9_1823b0535249  Port=11
  DiagcStsIvtr2Inactv : Inport  RequirementInfo={} %GIDa_6fd709e7_73cf_4f38_ab69_3c4606ea6b91  Port=12
  Trigger : TriggerPort  TriggerType=function-call  PortDimensions=1
  CopyRight2 : Subsystem  Description=|  mask(Copyright Information){none=on}
      | Copyright info block.                                               
      |                                                                     
      | Place copyright information at the top of every subsystem in design.
      mask prompts: none "No parameters"
      mask help: Place copyright information at the top of every subsystem in design.
      mask Display:
      | NxtrConf = 'Nexteer Confidential';
      | 
      | sys = bdroot; %handle for the current model ("system")
      | first = get_param(sys,'Created');
      | first = first(end-3:end);  %year is last four digits
      | 
      | last = get_param(sys,'LastModifiedDate');
      | if isempty(last)
      |     last = datestr(now,'yyyy');
      | else
      |     last = last(end-3:end);
      | end
      | 
      | if strcmp(first,last)
      |     fprintf('%s -- Copyright %s Nexteer',NxtrConf,first)
      | else
      |     fprintf('%s -- %s%s- %s Nexteer',NxtrConf,char(169),first,last)
      | end
  EolGainSt : DataStoreRead  DataStoreName=EolGainSts
  Gain Calibration : Subsystem  RequirementInfo={} %GIDa_dc55cc08_00d5_4d2c_9161_2782955335b3
  MotCurrEolCalStPrev : DataStoreWrite  RequirementInfo={} %GIDa_5bd07b1c_86e4_46fd_afdc_b357d0f0069c  DataStoreName=MotCurrEolCalStPrev  DataStoreElements=MotCurrEolCalStPrev
  Offset Calibration : Subsystem  RequirementInfo={} %GIDa_31f7e6d5_3bce_40cc_a784_8fd3d5abd669
  PIM1 : UnitDelay  SampleTime=-1  StateName=MotCurrOffsZeroAvrgA  StateMustResolveToSignalObject=on
      settings: AttributesFormatString=%<StateName>
  PIM2 : UnitDelay  SampleTime=-1  StateName=MotCurrOffsZeroAvrgB  StateMustResolveToSignalObject=on
      settings: AttributesFormatString=%<StateName>
  PIM3 : UnitDelay  SampleTime=-1  StateName=MotCurrOffsZeroAvrgC  StateMustResolveToSignalObject=on
      settings: AttributesFormatString=%<StateName>
  PIM4 : UnitDelay  SampleTime=-1  StateName=MotCurrOffsZeroAvrgD  StateMustResolveToSignalObject=on
      settings: AttributesFormatString=%<StateName>
  PIM5 : UnitDelay  SampleTime=-1  StateName=MotCurrOffsZeroAvrgE  StateMustResolveToSignalObject=on
      settings: AttributesFormatString=%<StateName>
  PIM6 : UnitDelay  SampleTime=-1  StateName=MotCurrOffsZeroAvrgF  StateMustResolveToSignalObject=on
      settings: AttributesFormatString=%<StateName>
  PIM7 : UnitDelay  SampleTime=-1  StateName=MotCurrEolOffsProcFlg  StateMustResolveToSignalObject=on
      settings: AttributesFormatString=%<StateName>
  Switch : Switch  Criteria=u2 > Threshold  OutDataTypeStr=Inherit: Inherit via back propagation
  MotCurrEolCalSt : Outport  RequirementInfo={} %GIDa_bd1a9dea_c496_413a_aa00_f3bf38f71498
  wires:
  Offset Calibration/2(MotCurrOffsZeroAvrgA) -> PIM1/1
  Offset Calibration/3(MotCurrOffsZeroAvrgB) -> PIM2/1
  Offset Calibration/4(MotCurrOffsZeroAvrgC) -> PIM3/1
  Offset Calibration/5(MotCurrOffsZeroAvrgD) -> PIM4/1
  Offset Calibration/6(MotCurrOffsZeroAvrgE) -> PIM5/1
  Offset Calibration/7(MotCurrOffsZeroAvrgF) -> PIM6/1
  Offset Calibration/1("MotCurrEolOffsProcFlg ") -> PIM7/1
  [VehSpd] -> Gain Calibration/15(VehSpd)
  [VehSpdVld] -> Gain Calibration/16(VehSpdVld)
  MotCurrAdcVlyA/1 -> Offset Calibration/1(In1), [MotCurrAdcVlyA]
  MotCurrAdcVlyC/1 -> [MotCurrAdcVlyC], Offset Calibration/3(In3)
  MotCurrAdcVlyE/1 -> [MotCurrAdcVlyE], Offset Calibration/5(In5)
  MotCurrAdcVlyD/1 -> [MotCurrAdcVlyD], Offset Calibration/4(In4)
  MotCurrAdcVlyB/1 -> [MotCurrAdcVlyB], Offset Calibration/2(In2)
  VehSpd/1 -> [VehSpd], Offset Calibration/9(VehSpd)
  BrdgVltg/1 -> Offset Calibration/8(In10)
  MotCurrAdcVlyF/1 -> [MotCurrAdcVlyF], Offset Calibration/6(In6)
  VehSpdVld/1 -> [VehSpdVld], Offset Calibration/10(VehSpdVld)
  MotVelMrf/1 -> [MotVelMrf], Offset Calibration/7(MotVelMrf)
  [MotCurrAdcVlyF] -> Gain Calibration/7(In6)
  [MotCurrAdcVlyB] -> Gain Calibration/3(In2)
  [MotCurrAdcVlyD] -> Gain Calibration/5(In4)
  [MotCurrAdcVlyE] -> Gain Calibration/6(In5)
  [MotCurrAdcVlyC] -> Gain Calibration/4(In3)
  [MotCurrAdcVlyA] -> Gain Calibration/2(In1)
  [MotVelMrf] -> Gain Calibration/8(MotVelMrf)
  PIM1/1 -> Gain Calibration/9(In11)
  PIM2/1 -> Gain Calibration/10(In12)
  PIM3/1 -> Gain Calibration/11(In13)
  PIM4/1 -> Gain Calibration/12(In14)
  PIM5/1 -> Gain Calibration/13(In15)
  PIM6/1 -> Gain Calibration/14(In16)
  PIM7/1 -> Gain Calibration/1(MotCurrEolOffsProcFlg)
  DiagcStsIvtr2Inactv/1 -> Gain Calibration/18(DiagcStsIvtr2Inactv), Offset Calibration/12(DiagcStsIvtr2Inactv)
  DiagcStsIvtr1Inactv/1 -> Gain Calibration/17(DiagcStsIvtr2Inactv1), Offset Calibration/11(DiagcStsIvtr1Inactv)
  Gain Calibration/1(CurrMeasMotCurrEolGainCalSt) -> Switch/1
  Offset Calibration/8(CurrMeasMotCurrEolOffsCalSt) -> Switch/3
  Switch/1 -> MotCurrEolCalStPrev/1, MotCurrEolCalSt/1
  EolGainSt/1 -> Switch/2
